simulink model "lab5_1"  (R2021a)
settings: Solver=VariableStepAuto  StartTime=0.0  StopTime=10.0  MaxStep=0.01  RelTol=1e-3
libraries: simulink_extras x1
settings Model: Creator=asr77  LastModifiedBy=asr77

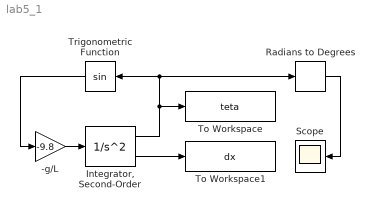
== system lab5_1 ==
  -g/L : Gain  Gain=-9.8
  "Integrator, Second-Order " : SecondOrderIntegrator  ICX=pi/100  ICDXDT=0
  "Radians to Degrees " : simulink_extras/Transformations/Radians to Degrees
  Scope : Scope
  To Workspace : ToWorkspace  VariableName=teta  SaveFormat=Timeseries  SampleTime=-1
      settings: Save2DSignal=2-D array (concatenate along first dimension)
  To Workspace1 : ToWorkspace  VariableName=dx  SaveFormat=Timeseries  SampleTime=-1
  "Trigonometric Function " : Trigonometry
  wires:
  "Integrator, Second-Order "/1 -> "Radians to Degrees "/1, "Trigonometric Function "/1, To Workspace/1
  "Trigonometric Function "/1 -> -g/L/1
  -g/L/1 -> "Integrator, Second-Order "/1
  "Radians to Degrees "/1 -> Scope/1
  "Integrator, Second-Order "/2 -> To Workspace1/1
